simulink model "InverterModel"  (R2016a)
settings: Solver=FixedStepDiscrete  StartTime=0.0  StopTime=0.55e-6  FixedStep=SampleTime  RelTol=1e-3
values from neighbouring files (symbols this model uses):
  DelayTop = 0    [InverterMFile.m]
  Dtop = 48    [InverterMFile.m]
  fsw = 2000e3    (= 2000000)    [InverterMFile.m]
  Rd = 0.0024 + 1e-4    (= 0.0025)    [InverterMFile.m]
  Rg = 1.5    [InverterMFile.m]
  Rload = 20    [InverterMFile.m]    (also in TwoLevelSPWM-Hakan.m = Zload*Load_Power_Factor)
  Roff = 2    [InverterMFile.m]
  Ron = 15    [InverterMFile.m]
  Rs = 0.0433 + 1e-4    (= 0.0434)    [InverterMFile.m]
  Rss = 1e-3    (= 0.001)    [InverterMFile.m]
  VpulseMax = 6    [InverterMFile.m]
  VpulseMin = -3    [InverterMFile.m]
libraries: elec_lib x129, nesl_utility x91, fl_lib x80, simulink x6
(part 5 of 5)

== system InverterModel/GAN HALF BRDIGE LEG2/GaN_Top1/Current Measure2 ==
  Current Sensor1 : fl_lib/Electrical/Electrical Sensors/Current Sensor
  PS-Simulink Converter4 : nesl_utility/PS-Simulink Converter  PhysicalDomain=network_engine_domain  SubClassName=ps_output  LeftPortType=input  RightPortType=output  PseudoPeriodic=off  Frequencies=[]  Unit=1  AffineConversion=off
  I+ : PMIOPort  Port=1  Side=Left
  I- : PMIOPort  Port=2  Side=Right
  Data : Outport
  wires:
  PS-Simulink Converter4/1 -> Data/1
  connections:
  Current Sensor1/RConn2 -- I-/RConn1
  PS-Simulink Converter4/LConn1 -- Current Sensor1/RConn1
  Current Sensor1/LConn1 -- I+/RConn1

== system InverterModel/GAN HALF BRDIGE LEG2/GaN_Top1/Current Measure3 ==
  Current Sensor1 : fl_lib/Electrical/Electrical Sensors/Current Sensor
  PS-Simulink Converter4 : nesl_utility/PS-Simulink Converter  PhysicalDomain=network_engine_domain  SubClassName=ps_output  LeftPortType=input  RightPortType=output  PseudoPeriodic=off  Frequencies=[]  Unit=1  AffineConversion=off
  I+ : PMIOPort  Port=1  Side=Left
  I- : PMIOPort  Port=2  Side=Right
  Data : Outport
  wires:
  PS-Simulink Converter4/1 -> Data/1
  connections:
  Current Sensor1/RConn2 -- I-/RConn1
  PS-Simulink Converter4/LConn1 -- Current Sensor1/RConn1
  Current Sensor1/LConn1 -- I+/RConn1

== system InverterModel/GAN HALF BRDIGE LEG2/GaN_Top1/Voltage Measure ==
  PS-Simulink Converter2 : nesl_utility/PS-Simulink Converter  PhysicalDomain=network_engine_domain  SubClassName=ps_output  LeftPortType=input  RightPortType=output  PseudoPeriodic=off  Frequencies=[]  Unit=1  AffineConversion=off
  Voltage Sensor3 : fl_lib/Electrical/Electrical Sensors/Voltage Sensor
  V+ : PMIOPort  Port=1  Side=Right
  V- : PMIOPort  Port=2  Side=Right
  Data : Outport
  wires:
  PS-Simulink Converter2/1 -> Data/1
  connections:
  PS-Simulink Converter2/LConn1 -- Voltage Sensor3/RConn1
  Voltage Sensor3/RConn2 -- V-/RConn1
  Voltage Sensor3/LConn1 -- V+/RConn1

== system InverterModel/GAN HALF BRDIGE LEG2/GaN_Top1/Voltage Measure1 ==
  PS-Simulink Converter2 : nesl_utility/PS-Simulink Converter  PhysicalDomain=network_engine_domain  SubClassName=ps_output  LeftPortType=input  RightPortType=output  PseudoPeriodic=off  Frequencies=[]  Unit=1  AffineConversion=off
  Voltage Sensor3 : fl_lib/Electrical/Electrical Sensors/Voltage Sensor
  V+ : PMIOPort  Port=1  Side=Right
  V- : PMIOPort  Port=2  Side=Right
  Data : Outport
  wires:
  PS-Simulink Converter2/1 -> Data/1
  connections:
  Voltage Sensor3/LConn1 -- V+/RConn1
  Voltage Sensor3/RConn2 -- V-/RConn1
  PS-Simulink Converter2/LConn1 -- Voltage Sensor3/RConn1

== system InverterModel/GAN HALF BRDIGE LEG2/GaN_Top1/Voltage Measure2 ==
  PS-Simulink Converter2 : nesl_utility/PS-Simulink Converter  PhysicalDomain=network_engine_domain  SubClassName=ps_output  LeftPortType=input  RightPortType=output  PseudoPeriodic=off  Frequencies=[]  Unit=1  AffineConversion=off
  Voltage Sensor3 : fl_lib/Electrical/Electrical Sensors/Voltage Sensor
  V+ : PMIOPort  Port=1  Side=Right
  V- : PMIOPort  Port=2  Side=Right
  Data : Outport
  wires:
  PS-Simulink Converter2/1 -> Data/1
  connections:
  PS-Simulink Converter2/LConn1 -- Voltage Sensor3/RConn1
  Voltage Sensor3/RConn2 -- V-/RConn1
  Voltage Sensor3/LConn1 -- V+/RConn1

== matlab function InverterModel/GAN HALF BRDIGE LEG1/GaN_Bot1/Capacitance Calculator1/MATLAB Function ==
  data: Vds input; Cgs output; Cgd output; Cds output; Vgs input
function [Cgs,Cgd,Cds]= fcn(Vds,Vgs)
%#codegen
% Vdc = 400;
% VpulseMax = 6;
% VpulseMin = -3;
% Vdsgs = (Vdc/(VpulseMax - VpulseMin))*(Vgs + VpulseMin);
Vds = abs(Vds);
%% Crss calculation
       a1 =   2.519e+14;
       b1 =      -345.7;
       c1 =       63.76;
       a2 =       27.99;
       b2 =       12.86;
       c2 =       18.29;
       a3 =       8.666;
       b3 =       33.93;
       c3 =       9.161;
       a4 =       1.502;
       b4 =       125.5;
       c4 =       121.9;
       a5 =      0.6563;
       b5 =         500;
       c5 =       34.57;
       a6 =        1.98;
       b6 =       408.2;
       c6 =       134.7;
Crss = a1.*exp(-((Vds-b1)./c1).^2) + a2.*exp(-((Vds-b2)./c2).^2) + a3*exp(-((Vds-b3)./c3).^2)...
   + a4.*exp(-((Vds-b4)./c4).^2) +a5.*exp(-((Vds-b5)./c5).^2) +a6.*exp(-((Vds-b6)./c6).^2);
Crss = Crss*1e-12;
%% Ciss Calculation
%        a1 =        1167;
%        b1 =      -115.8;
%        c1 =       60.96;
%        a2 =       269.7;
%        b2 =       -5402;
%        c2 =   4.243e+04;
%        a3 =        3.61;
%        b3 =       238.5;
%        c3 =       2.507;
%        a4 =       1.036;
%        b4 =       175.8;
%        c4 =       16.81;
%        a5 =       1.571;
%        b5 =         263;
%        c5 =       3.586;
%        a6 =      -1.174;
%        b6 =       238.2;
%        c6 =       25.85;
       a1 =        267.6;
       b1 =      2.007;
       c1 =       0.4734;
       a2 =       240.1;
       b2 =       3.049;
       c2 =      1.104;
       a3 =        -1336;
       b3 =       7.803;
       c3 =       9.331;
       a4 =       -250.6;
       b4 =       7.082;
       c4 =       1.715;
       a5 =       -2352;
       b5 =         11.25;
       c5 =       3.184;
       a6 =      8.572e13;
       b6 =       340.6;
       c6 =       67.72;
Ciss = a1.*exp(-((Vgs-b1)./c1).^2) + a2.*exp(-((Vgs-b2)./c2).^2) + a3*exp(-((Vgs-b3)./c3).^2)...
   + a4.*exp(-((Vgs-b4)./c4).^2) +a5.*exp(-((Vgs-b5)./c5).^2) +a6.*exp(-((Vgs-b6)./c6).^2);
Ciss = Ciss*1e-12;
%% Coss Calculation
       a1 =         328;
       b1 =       -8.43;
       c1 =       30.26;
       a2 =       115.8;
       b2 =        42.2;
       c2 =       7.341;
       a3 =       45.83;
       b3 =       59.01;
       c3 =       6.099;
       a4 =       183.1;
       b4 =        28.6;
       c4 =       16.39;
       a5 =       69.29;
       b5 =       154.4;
       c5 =        1511;
       a6 =       125.6;
       b6 =       22.68;
       c6 =       119.6;
Coss = a1.*exp(-((Vds-b1)./c1).^2) + a2.*exp(-((Vds-b2)./c2).^2) + a3*exp(-((Vds-b3)./c3).^2)...
   + a4.*exp(-((Vds-b4)./c4).^2) +a5.*exp(-((Vds-b5)./c5).^2) +a6.*exp(-((Vds-b6)./c6).^2);
Coss = Coss*1e-12;
%% Outputs
Cgs = Ciss - Crss;
Cds = Coss - Crss;
Cgd = Crss;

== matlab function InverterModel/GAN HALF BRDIGE LEG1/GaN_Bot1/MATLAB Function ==
  data: Vgs input; Ids output; Vds input
function Ids = fcn(Vgs,Vds)
%#codegen
% K1 = 0.283;
% b1 = 2.035;
% c1 = 0.124;
% d1 = 1.159;
% e1 = -0.204;
% m1 = 30.972;
% n1 = -4.48;
% K2 = 7.114;
% b2 = 2.054;
% c2 = 0.153;
Vgd = Vgs - Vds;

cur = 4.5057;
K = cur * 0.8 * (273/300)^(-2.7);
x0 = 0.31 ;
x1 = 0.255;
slp = 2;


% if Vds>0
%     Ids = K1*log(1+exp((Vgs-b1)/c1))*((m1+n1*Vgs)*Vds)/(1+(d1+e1*Vgs)*Vds);
% else
% 
%     Ids = -K2*log(1+exp((Vgd-b2)/c2))*(-Vds/(1-Vds));
% end

if Vds>0
    Ids = K*log(1+exp(26*(Vgs-1.7)/slp))*(Vds)/(1+max((x0+x1*(Vgs+4.1)),0.2)*Vds);
else

    Ids = -K*log(1+exp(21*(Vgd-1.7)/slp))*(-Vds)/(1+max((x0+x1*(Vgd+6.1)),0.2)*(-Vds));
end

== matlab function InverterModel/GAN HALF BRDIGE LEG1/GaN_Top1/Capacitance Calculator/MATLAB Function ==
  data: Vds input; Cgs output; Cgd output; Cds output; Vgs input
function [Cgs,Cgd,Cds]= fcn(Vds,Vgs)
%#codegen
% Vdc = 400;
% VpulseMax = 6;
% VpulseMin = -3;
% Vdsgs = (Vdc/(VpulseMax - VpulseMin))*(Vgs + VpulseMin);
Vds = abs(Vds);
%% Crss calculation
       a1 =   2.519e+14;
       b1 =      -345.7;
       c1 =       63.76;
       a2 =       27.99;
       b2 =       12.86;
       c2 =       18.29;
       a3 =       8.666;
       b3 =       33.93;
       c3 =       9.161;
       a4 =       1.502;
       b4 =       125.5;
       c4 =       121.9;
       a5 =      0.6563;
       b5 =         500;
       c5 =       34.57;
       a6 =        1.98;
       b6 =       408.2;
       c6 =       134.7;
Crss = a1.*exp(-((Vds-b1)./c1).^2) + a2.*exp(-((Vds-b2)./c2).^2) + a3*exp(-((Vds-b3)./c3).^2)...
   + a4.*exp(-((Vds-b4)./c4).^2) +a5.*exp(-((Vds-b5)./c5).^2) +a6.*exp(-((Vds-b6)./c6).^2);
Crss = Crss*1e-12;
%% Ciss Calculation
%        a1 =        1167;
%        b1 =      -115.8;
%        c1 =       60.96;
%        a2 =       269.7;
%        b2 =       -5402;
%        c2 =   4.243e+04;
%        a3 =        3.61;
%        b3 =       238.5;
%        c3 =       2.507;
%        a4 =       1.036;
%        b4 =       175.8;
%        c4 =       16.81;
%        a5 =       1.571;
%        b5 =         263;
%        c5 =       3.586;
%        a6 =      -1.174;
%        b6 =       238.2;
%        c6 =       25.85;
       a1 =        267.6;
       b1 =      2.007;
       c1 =       0.4734;
       a2 =       240.1;
       b2 =       3.049;
       c2 =      1.104;
       a3 =        -1336;
       b3 =       7.803;
       c3 =       9.331;
       a4 =       -250.6;
       b4 =       7.082;
       c4 =       1.715;
       a5 =       -2352;
       b5 =         11.25;
       c5 =       3.184;
       a6 =      8.572e13;
       b6 =       340.6;
       c6 =       67.72;
Ciss = a1.*exp(-((Vgs-b1)./c1).^2) + a2.*exp(-((Vgs-b2)./c2).^2) + a3*exp(-((Vgs-b3)./c3).^2)...
   + a4.*exp(-((Vgs-b4)./c4).^2) +a5.*exp(-((Vgs-b5)./c5).^2) +a6.*exp(-((Vgs-b6)./c6).^2);
Ciss = Ciss*1e-12;
%% Coss Calculation
       a1 =         328;
       b1 =       -8.43;
       c1 =       30.26;
       a2 =       115.8;
       b2 =        42.2;
       c2 =       7.341;
       a3 =       45.83;
       b3 =       59.01;
       c3 =       6.099;
       a4 =       183.1;
       b4 =        28.6;
       c4 =       16.39;
       a5 =       69.29;
       b5 =       154.4;
       c5 =        1511;
       a6 =       125.6;
       b6 =       22.68;
       c6 =       119.6;
Coss = a1.*exp(-((Vds-b1)./c1).^2) + a2.*exp(-((Vds-b2)./c2).^2) + a3*exp(-((Vds-b3)./c3).^2)...
   + a4.*exp(-((Vds-b4)./c4).^2) +a5.*exp(-((Vds-b5)./c5).^2) +a6.*exp(-((Vds-b6)./c6).^2);
Coss = Coss*1e-12;
%% Outputs
Cgs = Ciss - Crss;
Cds = Coss - Crss;
Cgd = Crss;

== matlab function InverterModel/GAN HALF BRDIGE LEG/GaN_Top1/Capacitance Calculator/MATLAB Function ==
  data: Vds input; Cgs output; Cgd output; Cds output; Vgs input
function [Cgs,Cgd,Cds]= fcn(Vds,Vgs)
%#codegen
% Vdc = 400;
% VpulseMax = 6;
% VpulseMin = -3;
% Vdsgs = (Vdc/(VpulseMax - VpulseMin))*(Vgs + VpulseMin);
Vds = abs(Vds);
%% Crss calculation
       a1 =   2.519e+14;
       b1 =      -345.7;
       c1 =       63.76;
       a2 =       27.99;
       b2 =       12.86;
       c2 =       18.29;
       a3 =       8.666;
       b3 =       33.93;
       c3 =       9.161;
       a4 =       1.502;
       b4 =       125.5;
       c4 =       121.9;
       a5 =      0.6563;
       b5 =         500;
       c5 =       34.57;
       a6 =        1.98;
       b6 =       408.2;
       c6 =       134.7;
Crss = a1.*exp(-((Vds-b1)./c1).^2) + a2.*exp(-((Vds-b2)./c2).^2) + a3*exp(-((Vds-b3)./c3).^2)...
   + a4.*exp(-((Vds-b4)./c4).^2) +a5.*exp(-((Vds-b5)./c5).^2) +a6.*exp(-((Vds-b6)./c6).^2);
Crss = Crss*1e-12;
%% Ciss Calculation
%        a1 =        1167;
%        b1 =      -115.8;
%        c1 =       60.96;
%        a2 =       269.7;
%        b2 =       -5402;
%        c2 =   4.243e+04;
%        a3 =        3.61;
%        b3 =       238.5;
%        c3 =       2.507;
%        a4 =       1.036;
%        b4 =       175.8;
%        c4 =       16.81;
%        a5 =       1.571;
%        b5 =         263;
%        c5 =       3.586;
%        a6 =      -1.174;
%        b6 =       238.2;
%        c6 =       25.85;
       a1 =        267.6;
       b1 =      2.007;
       c1 =       0.4734;
       a2 =       240.1;
       b2 =       3.049;
       c2 =      1.104;
       a3 =        -1336;
       b3 =       7.803;
       c3 =       9.331;
       a4 =       -250.6;
       b4 =       7.082;
       c4 =       1.715;
       a5 =       -2352;
       b5 =         11.25;
       c5 =       3.184;
       a6 =      8.572e13;
       b6 =       340.6;
       c6 =       67.72;
Ciss = a1.*exp(-((Vgs-b1)./c1).^2) + a2.*exp(-((Vgs-b2)./c2).^2) + a3*exp(-((Vgs-b3)./c3).^2)...
   + a4.*exp(-((Vgs-b4)./c4).^2) +a5.*exp(-((Vgs-b5)./c5).^2) +a6.*exp(-((Vgs-b6)./c6).^2);
Ciss = Ciss*1e-12;
%% Coss Calculation
       a1 =         328;
       b1 =       -8.43;
       c1 =       30.26;
       a2 =       115.8;
       b2 =        42.2;
       c2 =       7.341;
       a3 =       45.83;
       b3 =       59.01;
       c3 =       6.099;
       a4 =       183.1;
       b4 =        28.6;
       c4 =       16.39;
       a5 =       69.29;
       b5 =       154.4;
       c5 =        1511;
       a6 =       125.6;
       b6 =       22.68;
       c6 =       119.6;
Coss = a1.*exp(-((Vds-b1)./c1).^2) + a2.*exp(-((Vds-b2)./c2).^2) + a3*exp(-((Vds-b3)./c3).^2)...
   + a4.*exp(-((Vds-b4)./c4).^2) +a5.*exp(-((Vds-b5)./c5).^2) +a6.*exp(-((Vds-b6)./c6).^2);
Coss = Coss*1e-12;
%% Outputs
Cgs = Ciss - Crss;
Cds = Coss - Crss;
Cgd = Crss;

== matlab function InverterModel/Pulse Timing Block ==
  data: TopVA output; BotVA output; time input; TopVB output; BotVB output; TopVC output; BotVC output
function [TopVA,BotVA,TopVB,BotVB,TopVC,BotVC]= fcn(time)
fsw = 2000e3;
VpulseMax = 6;
VpulseMin = -3;
Dtop = 49; % duty cycle of top
Dbot = 49; % duty cycle of bot
% Phase Delays
DelayTopA = 0;
DelayBotA = 50;
DelayTopB = 100/3;
DelayBotB = 50 + 100/3;
DelayTopC = 200/3;
DelayBotC = 50 + 200/3 - 100;
% A Leg Gate Signals
PseudoTimeA = time;
while PseudoTimeA > 1/fsw
        PseudoTimeA = PseudoTimeA - 1/fsw;
end
    if (PseudoTimeA >= 0 && PseudoTimeA < (Dbot/100)/fsw) %bottom on top off dead time öncesi
        TopVA = VpulseMax;
        BotVA = VpulseMin;
   elseif (PseudoTimeA >= ((Dbot/100)/fsw) && PseudoTimeA < ((1-DelayBotA/100)/fsw))%bottom off oldu top off zaten dead time
        TopVA = VpulseMin;
        BotVA = VpulseMin;
    elseif PseudoTimeA >= ((DelayTopA/100)/fsw) && PseudoTimeA < ((0.5 + Dtop/100)/fsw) %% top on bottom off dead time öncesi
        TopVA = VpulseMin;
        BotVA = VpulseMax;
    else
        TopVA = VpulseMin;
        BotVA = VpulseMin;
    end
%B Leg Gate Signals
PseudoTimeB = 1/fsw - DelayTopB/100/fsw - PseudoTimeA;
while PseudoTimeB < 0
        PseudoTimeB = PseudoTimeB + 1/fsw;
end
    if (PseudoTimeB >= 0 && PseudoTimeB < (Dbot/100)/fsw) %bottom on top off dead time öncesi
        TopVB = VpulseMax;
        BotVB = VpulseMin;
   elseif (PseudoTimeB >= ((Dbot/100)/fsw) && PseudoTimeB < ((1-DelayBotA/100)/fsw))%bottom off oldu top off zaten dead time
        TopVB = VpulseMin;
        BotVB = VpulseMin;
    elseif PseudoTimeB >= ((DelayTopA/100)/fsw) && PseudoTimeB < ((0.5 + Dtop/100)/fsw) %% top on bottom off dead time öncesi
        TopVB = VpulseMin;
        BotVB = VpulseMax;
    else
        TopVB = VpulseMin;
        BotVB = VpulseMin;
    end
% C Leg Gate Signals
PseudoTimeC = 1/fsw - DelayTopC/100/fsw - PseudoTimeA;
while PseudoTimeC < 0
        PseudoTimeC = PseudoTimeC + 1/fsw;
end
    if (PseudoTimeC >= 0 && PseudoTimeC < (Dbot/100)/fsw) %bottom on top off dead time öncesi
        TopVC = VpulseMax;
        BotVC = VpulseMin;
   elseif (PseudoTimeC >= ((Dbot/100)/fsw) && PseudoTimeC < ((1-DelayBotA/100)/fsw))%bottom off oldu top off zaten dead time
        TopVC = VpulseMin;
        BotVC = VpulseMin;
    elseif PseudoTimeC >= ((DelayTopA/100)/fsw) && PseudoTimeC < ((0.5 + Dtop/100)/fsw) %% top on bottom off dead time öncesi
        TopVC = VpulseMin;
        BotVC = VpulseMax;
    else
        TopVC = VpulseMin;
        BotVC = VpulseMin;
    end

== matlab function InverterModel/GAN HALF BRDIGE LEG/GaN_Top1/MATLAB Function ==
  data: Vgs input; Ids output; Vds input
function Ids = fcn(Vgs,Vds)
%#codegen
% K1 = 0.283;
% b1 = 2.035;
% c1 = 0.124;
% d1 = 1.159;
% e1 = -0.204;
% m1 = 30.972;
% n1 = -4.48;
% K2 = 7.114;
% b2 = 2.054;
% c2 = 0.153;
% Vgs = 6;
% Vds = -0.045;
Vgd = Vgs - Vds;
cur = 4.5057;
K = cur * 0.8 * (273/300)^(-2.7);
x0 = 0.31 ;
x1 = 0.255;
slp = 2;


% if Vds>0
%     Ids = K1*log(1+exp((Vgs-b1)/c1))*((m1+n1*Vgs)*Vds)/(1+(d1+e1*Vgs)*Vds);
% else
% 
%     Ids = -K2*log(1+exp((Vgd-b2)/c2))*(-Vds/(1-Vds));
% end

if Vds>0
    Ids = K*log(1+exp(26*(Vgs-1.7)/slp))*(Vds)/(1+max((x0+x1*(Vgs+4.1)),0.2)*Vds);
else

    Ids = -K*log(1+exp(21*(Vgd-1.7)/slp))*(-Vds)/(1+max((x0+x1*(Vgd+6.1)),0.2)*(-Vds));
end

== matlab function InverterModel/GAN HALF BRDIGE LEG1/GaN_Top1/MATLAB Function ==
  data: Vgs input; Ids output; Vds input
function Ids = fcn(Vgs,Vds)
%#codegen
% K1 = 0.283;
% b1 = 2.035;
% c1 = 0.124;
% d1 = 1.159;
% e1 = -0.204;
% m1 = 30.972;
% n1 = -4.48;
% K2 = 7.114;
% b2 = 2.054;
% c2 = 0.153;
% Vgs = 6;
% Vds = -0.045;
Vgd = Vgs - Vds;
cur = 4.5057;
K = cur * 0.8 * (273/300)^(-2.7);
x0 = 0.31 ;
x1 = 0.255;
slp = 2;


% if Vds>0
%     Ids = K1*log(1+exp((Vgs-b1)/c1))*((m1+n1*Vgs)*Vds)/(1+(d1+e1*Vgs)*Vds);
% else
% 
%     Ids = -K2*log(1+exp((Vgd-b2)/c2))*(-Vds/(1-Vds));
% end

if Vds>0
    Ids = K*log(1+exp(26*(Vgs-1.7)/slp))*(Vds)/(1+max((x0+x1*(Vgs+4.1)),0.2)*Vds);
else

    Ids = -K*log(1+exp(21*(Vgd-1.7)/slp))*(-Vds)/(1+max((x0+x1*(Vgd+6.1)),0.2)*(-Vds));
end

== matlab function InverterModel/GAN HALF BRDIGE LEG/GaN_Bot1/Capacitance Calculator1/MATLAB Function ==
  data: Vds input; Cgs output; Cgd output; Cds output; Vgs input
function [Cgs,Cgd,Cds]= fcn(Vds,Vgs)
%#codegen
% Vdc = 400;
% VpulseMax = 6;
% VpulseMin = -3;
% Vdsgs = (Vdc/(VpulseMax - VpulseMin))*(Vgs + VpulseMin);
Vds = abs(Vds);
%% Crss calculation
       a1 =   2.519e+14;
       b1 =      -345.7;
       c1 =       63.76;
       a2 =       27.99;
       b2 =       12.86;
       c2 =       18.29;
       a3 =       8.666;
       b3 =       33.93;
       c3 =       9.161;
       a4 =       1.502;
       b4 =       125.5;
       c4 =       121.9;
       a5 =      0.6563;
       b5 =         500;
       c5 =       34.57;
       a6 =        1.98;
       b6 =       408.2;
       c6 =       134.7;
Crss = a1.*exp(-((Vds-b1)./c1).^2) + a2.*exp(-((Vds-b2)./c2).^2) + a3*exp(-((Vds-b3)./c3).^2)...
   + a4.*exp(-((Vds-b4)./c4).^2) +a5.*exp(-((Vds-b5)./c5).^2) +a6.*exp(-((Vds-b6)./c6).^2);
Crss = Crss*1e-12;
%% Ciss Calculation
%        a1 =        1167;
%        b1 =      -115.8;
%        c1 =       60.96;
%        a2 =       269.7;
%        b2 =       -5402;
%        c2 =   4.243e+04;
%        a3 =        3.61;
%        b3 =       238.5;
%        c3 =       2.507;
%        a4 =       1.036;
%        b4 =       175.8;
%        c4 =       16.81;
%        a5 =       1.571;
%        b5 =         263;
%        c5 =       3.586;
%        a6 =      -1.174;
%        b6 =       238.2;
%        c6 =       25.85;
       a1 =        267.6;
       b1 =      2.007;
       c1 =       0.4734;
       a2 =       240.1;
       b2 =       3.049;
       c2 =      1.104;
       a3 =        -1336;
       b3 =       7.803;
       c3 =       9.331;
       a4 =       -250.6;
       b4 =       7.082;
       c4 =       1.715;
       a5 =       -2352;
       b5 =         11.25;
       c5 =       3.184;
       a6 =      8.572e13;
       b6 =       340.6;
       c6 =       67.72;
Ciss = a1.*exp(-((Vgs-b1)./c1).^2) + a2.*exp(-((Vgs-b2)./c2).^2) + a3*exp(-((Vgs-b3)./c3).^2)...
   + a4.*exp(-((Vgs-b4)./c4).^2) +a5.*exp(-((Vgs-b5)./c5).^2) +a6.*exp(-((Vgs-b6)./c6).^2);
Ciss = Ciss*1e-12;
%% Coss Calculation
       a1 =         328;
       b1 =       -8.43;
       c1 =       30.26;
       a2 =       115.8;
       b2 =        42.2;
       c2 =       7.341;
       a3 =       45.83;
       b3 =       59.01;
       c3 =       6.099;
       a4 =       183.1;
       b4 =        28.6;
       c4 =       16.39;
       a5 =       69.29;
       b5 =       154.4;
       c5 =        1511;
       a6 =       125.6;
       b6 =       22.68;
       c6 =       119.6;
Coss = a1.*exp(-((Vds-b1)./c1).^2) + a2.*exp(-((Vds-b2)./c2).^2) + a3*exp(-((Vds-b3)./c3).^2)...
   + a4.*exp(-((Vds-b4)./c4).^2) +a5.*exp(-((Vds-b5)./c5).^2) +a6.*exp(-((Vds-b6)./c6).^2);
Coss = Coss*1e-12;
%% Outputs
Cgs = Ciss - Crss;
Cds = Coss - Crss;
Cgd = Crss;

== matlab function InverterModel/GAN HALF BRDIGE LEG/GaN_Bot1/MATLAB Function ==
  data: Vgs input; Ids output; Vds input
function Ids = fcn(Vgs,Vds)
%#codegen
% K1 = 0.283;
% b1 = 2.035;
% c1 = 0.124;
% d1 = 1.159;
% e1 = -0.204;
% m1 = 30.972;
% n1 = -4.48;
% K2 = 7.114;
% b2 = 2.054;
% c2 = 0.153;
Vgd = Vgs - Vds;

cur = 4.5057;
K = cur * 0.8 * (273/300)^(-2.7);
x0 = 0.31 ;
x1 = 0.255;
slp = 2;


% if Vds>0
%     Ids = K1*log(1+exp((Vgs-b1)/c1))*((m1+n1*Vgs)*Vds)/(1+(d1+e1*Vgs)*Vds);
% else
% 
%     Ids = -K2*log(1+exp((Vgd-b2)/c2))*(-Vds/(1-Vds));
% end

if Vds>0
    Ids = K*log(1+exp(26*(Vgs-1.7)/slp))*(Vds)/(1+max((x0+x1*(Vgs+4.1)),0.2)*Vds);
else

    Ids = -K*log(1+exp(21*(Vgd-1.7)/slp))*(-Vds)/(1+max((x0+x1*(Vgd+6.1)),0.2)*(-Vds));
end

== matlab function InverterModel/GAN HALF BRDIGE LEG2/GaN_Bot1/Capacitance Calculator1/MATLAB Function ==
  data: Vds input; Cgs output; Cgd output; Cds output; Vgs input
function [Cgs,Cgd,Cds]= fcn(Vds,Vgs)
%#codegen
% Vdc = 400;
% VpulseMax = 6;
% VpulseMin = -3;
% Vdsgs = (Vdc/(VpulseMax - VpulseMin))*(Vgs + VpulseMin);
Vds = abs(Vds);
%% Crss calculation
       a1 =   2.519e+14;
       b1 =      -345.7;
       c1 =       63.76;
       a2 =       27.99;
       b2 =       12.86;
       c2 =       18.29;
       a3 =       8.666;
       b3 =       33.93;
       c3 =       9.161;
       a4 =       1.502;
       b4 =       125.5;
       c4 =       121.9;
       a5 =      0.6563;
       b5 =         500;
       c5 =       34.57;
       a6 =        1.98;
       b6 =       408.2;
       c6 =       134.7;
Crss = a1.*exp(-((Vds-b1)./c1).^2) + a2.*exp(-((Vds-b2)./c2).^2) + a3*exp(-((Vds-b3)./c3).^2)...
   + a4.*exp(-((Vds-b4)./c4).^2) +a5.*exp(-((Vds-b5)./c5).^2) +a6.*exp(-((Vds-b6)./c6).^2);
Crss = Crss*1e-12;
%% Ciss Calculation
%        a1 =        1167;
%        b1 =      -115.8;
%        c1 =       60.96;
%        a2 =       269.7;
%        b2 =       -5402;
%        c2 =   4.243e+04;
%        a3 =        3.61;
%        b3 =       238.5;
%        c3 =       2.507;
%        a4 =       1.036;
%        b4 =       175.8;
%        c4 =       16.81;
%        a5 =       1.571;
%        b5 =         263;
%        c5 =       3.586;
%        a6 =      -1.174;
%        b6 =       238.2;
%        c6 =       25.85;
       a1 =        267.6;
       b1 =      2.007;
       c1 =       0.4734;
       a2 =       240.1;
       b2 =       3.049;
       c2 =      1.104;
       a3 =        -1336;
       b3 =       7.803;
       c3 =       9.331;
       a4 =       -250.6;
       b4 =       7.082;
       c4 =       1.715;
       a5 =       -2352;
       b5 =         11.25;
       c5 =       3.184;
       a6 =      8.572e13;
       b6 =       340.6;
       c6 =       67.72;
Ciss = a1.*exp(-((Vgs-b1)./c1).^2) + a2.*exp(-((Vgs-b2)./c2).^2) + a3*exp(-((Vgs-b3)./c3).^2)...
   + a4.*exp(-((Vgs-b4)./c4).^2) +a5.*exp(-((Vgs-b5)./c5).^2) +a6.*exp(-((Vgs-b6)./c6).^2);
Ciss = Ciss*1e-12;
%% Coss Calculation
       a1 =         328;
       b1 =       -8.43;
       c1 =       30.26;
       a2 =       115.8;
       b2 =        42.2;
       c2 =       7.341;
       a3 =       45.83;
       b3 =       59.01;
       c3 =       6.099;
       a4 =       183.1;
       b4 =        28.6;
       c4 =       16.39;
       a5 =       69.29;
       b5 =       154.4;
       c5 =        1511;
       a6 =       125.6;
       b6 =       22.68;
       c6 =       119.6;
Coss = a1.*exp(-((Vds-b1)./c1).^2) + a2.*exp(-((Vds-b2)./c2).^2) + a3*exp(-((Vds-b3)./c3).^2)...
   + a4.*exp(-((Vds-b4)./c4).^2) +a5.*exp(-((Vds-b5)./c5).^2) +a6.*exp(-((Vds-b6)./c6).^2);
Coss = Coss*1e-12;
%% Outputs
Cgs = Ciss - Crss;
Cds = Coss - Crss;
Cgd = Crss;

== matlab function InverterModel/GAN HALF BRDIGE LEG2/GaN_Bot1/MATLAB Function ==
  data: Vgs input; Ids output; Vds input
function Ids = fcn(Vgs,Vds)
%#codegen
% K1 = 0.283;
% b1 = 2.035;
% c1 = 0.124;
% d1 = 1.159;
% e1 = -0.204;
% m1 = 30.972;
% n1 = -4.48;
% K2 = 7.114;
% b2 = 2.054;
% c2 = 0.153;
Vgd = Vgs - Vds;

cur = 4.5057;
K = cur * 0.8 * (273/300)^(-2.7);
x0 = 0.31 ;
x1 = 0.255;
slp = 2;


% if Vds>0
%     Ids = K1*log(1+exp((Vgs-b1)/c1))*((m1+n1*Vgs)*Vds)/(1+(d1+e1*Vgs)*Vds);
% else
% 
%     Ids = -K2*log(1+exp((Vgd-b2)/c2))*(-Vds/(1-Vds));
% end

if Vds>0
    Ids = K*log(1+exp(26*(Vgs-1.7)/slp))*(Vds)/(1+max((x0+x1*(Vgs+4.1)),0.2)*Vds);
else

    Ids = -K*log(1+exp(21*(Vgd-1.7)/slp))*(-Vds)/(1+max((x0+x1*(Vgd+6.1)),0.2)*(-Vds));
end

== matlab function InverterModel/GAN HALF BRDIGE LEG2/GaN_Top1/Capacitance Calculator/MATLAB Function ==
  data: Vds input; Cgs output; Cgd output; Cds output; Vgs input
function [Cgs,Cgd,Cds]= fcn(Vds,Vgs)
%#codegen
% Vdc = 400;
% VpulseMax = 6;
% VpulseMin = -3;
% Vdsgs = (Vdc/(VpulseMax - VpulseMin))*(Vgs + VpulseMin);
Vds = abs(Vds);
%% Crss calculation
       a1 =   2.519e+14;
       b1 =      -345.7;
       c1 =       63.76;
       a2 =       27.99;
       b2 =       12.86;
       c2 =       18.29;
       a3 =       8.666;
       b3 =       33.93;
       c3 =       9.161;
       a4 =       1.502;
       b4 =       125.5;
       c4 =       121.9;
       a5 =      0.6563;
       b5 =         500;
       c5 =       34.57;
       a6 =        1.98;
       b6 =       408.2;
       c6 =       134.7;
Crss = a1.*exp(-((Vds-b1)./c1).^2) + a2.*exp(-((Vds-b2)./c2).^2) + a3*exp(-((Vds-b3)./c3).^2)...
   + a4.*exp(-((Vds-b4)./c4).^2) +a5.*exp(-((Vds-b5)./c5).^2) +a6.*exp(-((Vds-b6)./c6).^2);
Crss = Crss*1e-12;
%% Ciss Calculation
%        a1 =        1167;
%        b1 =      -115.8;
%        c1 =       60.96;
%        a2 =       269.7;
%        b2 =       -5402;
%        c2 =   4.243e+04;
%        a3 =        3.61;
%        b3 =       238.5;
%        c3 =       2.507;
%        a4 =       1.036;
%        b4 =       175.8;
%        c4 =       16.81;
%        a5 =       1.571;
%        b5 =         263;
%        c5 =       3.586;
%        a6 =      -1.174;
%        b6 =       238.2;
%        c6 =       25.85;
       a1 =        267.6;
       b1 =      2.007;
       c1 =       0.4734;
       a2 =       240.1;
       b2 =       3.049;
       c2 =      1.104;
       a3 =        -1336;
       b3 =       7.803;
       c3 =       9.331;
       a4 =       -250.6;
       b4 =       7.082;
       c4 =       1.715;
       a5 =       -2352;
       b5 =         11.25;
       c5 =       3.184;
       a6 =      8.572e13;
       b6 =       340.6;
       c6 =       67.72;
Ciss = a1.*exp(-((Vgs-b1)./c1).^2) + a2.*exp(-((Vgs-b2)./c2).^2) + a3*exp(-((Vgs-b3)./c3).^2)...
   + a4.*exp(-((Vgs-b4)./c4).^2) +a5.*exp(-((Vgs-b5)./c5).^2) +a6.*exp(-((Vgs-b6)./c6).^2);
Ciss = Ciss*1e-12;
%% Coss Calculation
       a1 =         328;
       b1 =       -8.43;
       c1 =       30.26;
       a2 =       115.8;
       b2 =        42.2;
       c2 =       7.341;
       a3 =       45.83;
       b3 =       59.01;
       c3 =       6.099;
       a4 =       183.1;
       b4 =        28.6;
       c4 =       16.39;
       a5 =       69.29;
       b5 =       154.4;
       c5 =        1511;
       a6 =       125.6;
       b6 =       22.68;
       c6 =       119.6;
Coss = a1.*exp(-((Vds-b1)./c1).^2) + a2.*exp(-((Vds-b2)./c2).^2) + a3*exp(-((Vds-b3)./c3).^2)...
   + a4.*exp(-((Vds-b4)./c4).^2) +a5.*exp(-((Vds-b5)./c5).^2) +a6.*exp(-((Vds-b6)./c6).^2);
Coss = Coss*1e-12;
%% Outputs
Cgs = Ciss - Crss;
Cds = Coss - Crss;
Cgd = Crss;

== matlab function InverterModel/GAN HALF BRDIGE LEG2/GaN_Top1/MATLAB Function ==
  data: Vgs input; Ids output; Vds input
function Ids = fcn(Vgs,Vds)
%#codegen
% K1 = 0.283;
% b1 = 2.035;
% c1 = 0.124;
% d1 = 1.159;
% e1 = -0.204;
% m1 = 30.972;
% n1 = -4.48;
% K2 = 7.114;
% b2 = 2.054;
% c2 = 0.153;
% Vgs = 6;
% Vds = -0.045;
Vgd = Vgs - Vds;
cur = 4.5057;
K = cur * 0.8 * (273/300)^(-2.7);
x0 = 0.31 ;
x1 = 0.255;
slp = 2;


% if Vds>0
%     Ids = K1*log(1+exp((Vgs-b1)/c1))*((m1+n1*Vgs)*Vds)/(1+(d1+e1*Vgs)*Vds);
% else
% 
%     Ids = -K2*log(1+exp((Vgd-b2)/c2))*(-Vds/(1-Vds));
% end

if Vds>0
    Ids = K*log(1+exp(26*(Vgs-1.7)/slp))*(Vds)/(1+max((x0+x1*(Vgs+4.1)),0.2)*Vds);
else

    Ids = -K*log(1+exp(21*(Vgd-1.7)/slp))*(-Vds)/(1+max((x0+x1*(Vgd+6.1)),0.2)*(-Vds));
end
